simulink model "test_nncLKAsys"  (R2023a)
settings: Solver=VariableStepAuto  StartTime=0.0  StopTime=15  RelTol=1e-3
undefined symbols (not defined in the file): Cf, Cr, Iz, lf, lr, m, md, Ts, Vx
libraries: neural x49
(part 2 of 2)

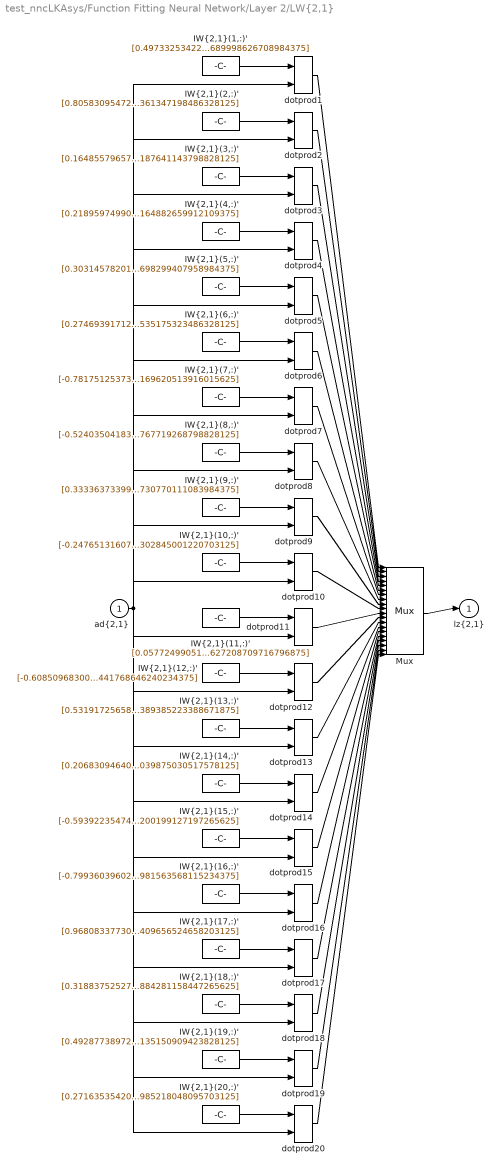
== system test_nncLKAsys/Function Fitting Neural Network/Layer 2/LW{2,1} ==
  "ad{2,1}" : Inport  PortDimensions=20
      mask Display: e = 0.06;c1 = [120 230 180]/255;c2 = ([120 230 180]+0)/(256+128);c3 = ([120 230 180]+128)/(256+128);patch([0 1 1 0],[0 0 1 1],c1);patch([0 1 1 1-e 1-e 0+e],[0 0 1 1-e 0+e 0+e],c2);patch([0 0 1 1-e 0+e 0+e],[0 1 1 1-e 1-e 0+e],c3);plot([0 1 1 0 0],[0 0 1 1 0]);
  "IW{2,1}(1,:)'" : Constant  Value=[0.4973325342225560774522818974219262599945068359375;0.90306464526148644278435995147447101771831512451171875;-0.496048746421447861454367966871359385550022125244140625;0.86588830289279539176305888759088702499866485595703125;0.258362950744856101348290167152299545705318450927734375;-0.7205856953057050429123364665429107844829559326171875;0.6406037637494745862198897157213650643825531005859375;0.054448589267391871160395311335378210060298442840576171875;0.05120315605558094229632359883908065967261791229248046875;0.734496230646326520030697793117724359035491943359375;0.440526641299326338074848763426416553556919097900390625;-0.443526764242088145095976869924925267696380615234375;-0.124610565537413064962635189658612944185733795166015625;0.495622454954692204243116293582716025412082672119140625;-0.274663451448240447660964491660706698894500732421875;-0.95942325063411926233669646535417996346950531005859375;-0.4074690282329813673101170934387482702732086181640625;-0.3830663272716934297790203345357440412044525146484375;0.37164147603418851151246826702845282852649688720703125;-0.418196849214901023028545523629873059689998626708984375]
      mask Display: e = 0.06;c1 = [120 150 230]/255;c2 = ([120 150 230]+0)/383;c3 = ([120 150 230]+128)/383;patch([0 1 1 0],[0 0 1 1],c1);patch([0 1 1 1-e 1-e 0+e],[0 0 1 1-e 0+e 0+e],c2);patch([0 0 1 1-e 0+e 0+e],[0 1 1 1-e 1-e 0+e],c3);plot([0 1 1 0 0],[0 0 1 1 0]);disp('weights');
  "IW{2,1}(10,:)'" : Constant  Value=[-0.2476513160780807465410902068470022641122341156005859375;-0.05048981524499081274814926700855721719563007354736328125;-0.83187777564385922968170916647068224847316741943359375;-0.1842943675353526378213331327060586772859096527099609375;-0.135408743923043306534026442022877745330333709716796875;0.213378955593828967263192453174269758164882659912109375;0.291693823371609373129587083894875831902027130126953125;-0.463136288082497682427884910794091410934925079345703125;-0.2209047101854656747210725598051794804632663726806640625;0.47999229837702539480659424953046254813671112060546875;0.70943574543465448556389674195088446140289306640625;-0.822960664207583736384776784689165651798248291015625;0.46371966171671552547906003383104689419269561767578125;0.35777426056320293934476239883224479854106903076171875;-0.053457236318613009229405719224814674817025661468505859375;-0.5644419341845097193299807258881628513336181640625;-0.830852975041227903574281299370341002941131591796875;-0.8407291227819257972697641889681108295917510986328125;-0.9051254349425936762685296343988738954067230224609375;-0.51676331967606270456627726161968894302845001220703125]
      mask Display: e = 0.06;c1 = [120 150 230]/255;c2 = ([120 150 230]+0)/383;c3 = ([120 150 230]+128)/383;patch([0 1 1 0],[0 0 1 1],c1);patch([0 1 1 1-e 1-e 0+e],[0 0 1 1-e 0+e 0+e],c2);patch([0 0 1 1-e 0+e 0+e],[0 1 1 1-e 1-e 0+e],c3);plot([0 1 1 0 0],[0 0 1 1 0]);disp('weights');
  "IW{2,1}(11,:)'" : Constant  Value=[0.057724990515373324206915839340581442229449748992919921875;-0.454959352688771134776146709555177949368953704833984375;0.686013523400408331553990137763321399688720703125;0.77761666694430864321674334860290400683879852294921875;-0.67233436458554962644740271571208722889423370361328125;0.262387251003185772990633495282963849604129791259765625;0.66393479253179810140039762700325809419155120849609375;-0.54205992204004826984231613096198998391628265380859375;0.659601736923068671103465021587908267974853515625;0.59560282814388243455283600269467569887638092041015625;-0.67025312054929220284549273856100626289844512939453125;-0.0109594114292667112187107392173857078887522220611572265625;0.1323308886400174078090685725328512489795684814453125;0.77709052240416143231271917102276347577571868896484375;-0.272148319240205383007236150660901330411434173583984375;0.59914332019493798942022522169281728565692901611328125;0.99457188770306415026567492532194592058658599853515625;0.37686351449791433143587937593110837042331695556640625;0.616532923458239512370937518426217138767242431640625;-0.3508767302809150390174863787251524627208709716796875]
      mask Display: e = 0.06;c1 = [120 150 230]/255;c2 = ([120 150 230]+0)/383;c3 = ([120 150 230]+128)/383;patch([0 1 1 0],[0 0 1 1],c1);patch([0 1 1 1-e 1-e 0+e],[0 0 1 1-e 0+e 0+e],c2);patch([0 0 1 1-e 0+e 0+e],[0 1 1 1-e 1-e 0+e],c3);plot([0 1 1 0 0],[0 0 1 1 0]);disp('weights');
  "IW{2,1}(12,:)'" : Constant  Value=[-0.60850968300268626354210255158250220119953155517578125;-0.65439626701131403674338571363477967679500579833984375;0.402047200135600302228766622647526673972606658935546875;0.3978796710819414439441743525094352662563323974609375;0.36291812080822760666620752090238966047763824462890625;0.4909388105689107550944072499987669289112091064453125;-0.480859970862364261012800170647096820175647735595703125;0.26633703325919200199933811745722778141498565673828125;-0.67734265099850732294584076953469775617122650146484375;-0.246990874667310122969610119980643503367900848388671875;-0.0149495709028309962940195276814847602508962154388427734375;0.85590287991131053235704939652350731194019317626953125;-0.52043442213506352356233719547162763774394989013671875;-0.72331221909417309223755410130252130329608917236328125;-0.72319113937276202630499710721778683364391326904296875;0.27801325599222603823790223032119683921337127685546875;-0.720583773337928779056937855784781277179718017578125;0.7117053121012466565531440210179425776004791259765625;0.19320449486644986070160712188226170837879180908203125;-0.55058864749936853311140794176026247441768646240234375]
      mask Display: e = 0.06;c1 = [120 150 230]/255;c2 = ([120 150 230]+0)/383;c3 = ([120 150 230]+128)/383;patch([0 1 1 0],[0 0 1 1],c1);patch([0 1 1 1-e 1-e 0+e],[0 0 1 1-e 0+e 0+e],c2);patch([0 0 1 1-e 0+e 0+e],[0 1 1 1-e 1-e 0+e],c3);plot([0 1 1 0 0],[0 0 1 1 0]);disp('weights');
  "IW{2,1}(13,:)'" : Constant  Value=[0.53191725658587396541321368204080499708652496337890625;-0.5684191622120613462953997441218234598636627197265625;0.21829186796840016615561808066559024155139923095703125;0.8434716025869997135799849274917505681514739990234375;-0.429187862165322064900152554400847293436527252197265625;-0.61841840572703576928148549995967186987400054931640625;0.6095584518567715992531930169207043945789337158203125;-0.276179360087225822528722574134008027613162994384765625;0.2433613583566199556340592380365706048905849456787109375;0.98001673052718574208341806297539733350276947021484375;-0.45880540181842321967309317187755368649959564208984375;0.06691757909025740358455180967212072573602199554443359375;-0.7740737648085611599668709459365345537662506103515625;0.8386821929981544965215789488865993916988372802734375;-0.76226447852808776328714657211094163358211517333984375;0.5511304110054016103248386571067385375499725341796875;0.239317115231703070321600534953176975250244140625;-0.75148183567851145614469032807392068207263946533203125;-0.475776517023930589633806675919913686811923980712890625;-0.65629454419391464181643414121936075389385223388671875]
      mask Display: e = 0.06;c1 = [120 150 230]/255;c2 = ([120 150 230]+0)/383;c3 = ([120 150 230]+128)/383;patch([0 1 1 0],[0 0 1 1],c1);patch([0 1 1 1-e 1-e 0+e],[0 0 1 1-e 0+e 0+e],c2);patch([0 0 1 1-e 0+e 0+e],[0 1 1 1-e 1-e 0+e],c3);plot([0 1 1 0 0],[0 0 1 1 0]);disp('weights');
  "IW{2,1}(14,:)'" : Constant  Value=[0.2068309464048300461147533724215463735163211822509765625;-0.060874669609953351023801104702215525321662425994873046875;0.042469111138720129494661392755006090737879276275634765625;0.75101380689437513549222558140172623097896575927734375;-0.2301884916521317325788231755723245441913604736328125;-0.64214453268418092424241194748901762068271636962890625;-0.37040855858182430981884181164787150919437408447265625;-0.70737191728260040424203225484234280884265899658203125;-0.135073111944455648281149251488386653363704681396484375;1.0030017572738476605564983401563949882984161376953125;0.554473075215879962485132637084461748600006103515625;-0.5767995535584378163918017889955081045627593994140625;-0.10154501148795087861476105217661825008690357208251953125;0.83011392912038461933121880065300501883029937744140625;-0.022470298944575924082744933230060269124805927276611328125;0.484985641342478512871849716248107142746448516845703125;-0.1963460027903477234101359272244735620915889739990234375;-0.261489162470172953334213161724619567394256591796875;0.88801671382668134757665256984182633459568023681640625;0.8012075193285348451155414295499213039875030517578125]
      mask Display: e = 0.06;c1 = [120 150 230]/255;c2 = ([120 150 230]+0)/383;c3 = ([120 150 230]+128)/383;patch([0 1 1 0],[0 0 1 1],c1);patch([0 1 1 1-e 1-e 0+e],[0 0 1 1-e 0+e 0+e],c2);patch([0 0 1 1-e 0+e 0+e],[0 1 1 1-e 1-e 0+e],c3);plot([0 1 1 0 0],[0 0 1 1 0]);disp('weights');
  "IW{2,1}(15,:)'" : Constant  Value=[-0.59392235474925125782164059273782186210155487060546875;0.2469970517320487501944370478668133728206157684326171875;-0.479182699839034775823876088907127268612384796142578125;-0.7565554149826076990592582660610787570476531982421875;-0.147267538182649870837082062280387617647647857666015625;-1.101355612636625291855807518004439771175384521484375;0.414661477953157830977914954928564839065074920654296875;-0.57924333285030626949918541868100874125957489013671875;-0.2822483427932775956747946111136116087436676025390625;0.365463041905304153456057747462182305753231048583984375;0.691449731034453396461003649164922535419464111328125;-0.484014696014661460754524568983470089733600616455078125;-0.3214298163255582263531096032238565385341644287109375;-0.2446932497166434961055614394354051910340785980224609375;0.87806342417053884208399949784507043659687042236328125;-0.6837950072062544126794136900571174919605255126953125;-0.1294637551593125490700941782051813788712024688720703125;-0.51639178539500318887434104908606968820095062255859375;-0.8628656967513392839208563600550405681133270263671875;0.57210024503377587823393923827097751200199127197265625]
      mask Display: e = 0.06;c1 = [120 150 230]/255;c2 = ([120 150 230]+0)/383;c3 = ([120 150 230]+128)/383;patch([0 1 1 0],[0 0 1 1],c1);patch([0 1 1 1-e 1-e 0+e],[0 0 1 1-e 0+e 0+e],c2);patch([0 0 1 1-e 0+e 0+e],[0 1 1 1-e 1-e 0+e],c3);plot([0 1 1 0 0],[0 0 1 1 0]);disp('weights');
  "IW{2,1}(16,:)'" : Constant  Value=[-0.79936039602108255319734553268062882125377655029296875;-0.9038848231317271331164420189452357590198516845703125;0.404706321969310167663280708438833244144916534423828125;0.369308486120014212161777322762645781040191650390625;-0.73588945289850615782967224731692112982273101806640625;0.2109720089806362552931062737116008065640926361083984375;0.80563130849964437185661836338113062083721160888671875;0.173851749513278586167785988436662591993808746337890625;-0.2151500541783762654457490270942798815667629241943359375;0.408657702026222369173780180062749423086643218994140625;-0.9027615049856836382247138317325152456760406494140625;0.0172054680890415361005363337199014495126903057098388671875;-0.8622846305143279099780784235917963087558746337890625;-0.51387189745748995672869341433397494256496429443359375;-0.55544867935312336459929838383686728775501251220703125;0.3756122611517251907997660964610986411571502685546875;0.553092246700364942313399296835996210575103759765625;-0.84888335556626592914852835747296921908855438232421875;-0.8758198815178668272807271932833828032016754150390625;0.74301445501374396851446135769947431981563568115234375]
      mask Display: e = 0.06;c1 = [120 150 230]/255;c2 = ([120 150 230]+0)/383;c3 = ([120 150 230]+128)/383;patch([0 1 1 0],[0 0 1 1],c1);patch([0 1 1 1-e 1-e 0+e],[0 0 1 1-e 0+e 0+e],c2);patch([0 0 1 1-e 0+e 0+e],[0 1 1 1-e 1-e 0+e],c3);plot([0 1 1 0 0],[0 0 1 1 0]);disp('weights');
  "IW{2,1}(17,:)'" : Constant  Value=[0.96808337730736437887202328056446276605129241943359375;0.8804707813004741812079601004370488226413726806640625;0.102363658179670580228304288539220578968524932861328125;-0.8352226572803538306999371343408711254596710205078125;0.9505108042221801500915034921490587294101715087890625;0.438235898788289002236950864244136027991771697998046875;0.38577234970647855671899151275283657014369964599609375;-0.1208143097052460090967684891438693739473819732666015625;-0.77150614240208081895389113924466073513031005859375;0.84947514259350132004300348853575997054576873779296875;-0.1487735383250336218541320931763038970530033111572265625;0.87542171746614150240617391318664886057376861572265625;-0.94090955821116850632535033582826144993305206298828125;-0.89715669844669954091642694038455374538898468017578125;-0.81592915906335949927097317413426935672760009765625;0.492156990589912857192445017062709666788578033447265625;0.08283113566716497622177683979316498152911663055419921875;-0.488791100114578214164140490538557060062885284423828125;0.2348206770858200786999958609158056788146495819091796875;0.59500478527796485384016023090225644409656524658203125]
      mask Display: e = 0.06;c1 = [120 150 230]/255;c2 = ([120 150 230]+0)/383;c3 = ([120 150 230]+128)/383;patch([0 1 1 0],[0 0 1 1],c1);patch([0 1 1 1-e 1-e 0+e],[0 0 1 1-e 0+e 0+e],c2);patch([0 0 1 1-e 0+e 0+e],[0 1 1 1-e 1-e 0+e],c3);plot([0 1 1 0 0],[0 0 1 1 0]);disp('weights');
  "IW{2,1}(18,:)'" : Constant  Value=[0.318837525273336808151469767835806123912334442138671875;-0.0466292350120939003144115986287943087518215179443359375;0.74492191849115896307154116584570147097110748291015625;1.0461389061517232246245612259372137486934661865234375;0.8703366566824921601863707110169343650341033935546875;0.807666727616154656033131686854176223278045654296875;-0.79258773942038052151559668345726095139980316162109375;0.00021271701060131438520972579908629995770752429962158203125;0.811323814918487595804208467598073184490203857421875;-0.8942994208564523095361664672964252531528472900390625;0.704688427044971366086656416882760822772979736328125;-1.0132738674596739603117612205096520483493804931640625;0.30231916343964126969723338334006257355213165283203125;0.81174905074590653075716772946179844439029693603515625;-0.0025264614549911266171144941239390391274355351924896240234375;-0.33930147473698590854240819680853746831417083740234375;-0.1348439869058445095273413016911945305764675140380859375;-0.60934272120341559375589213232160545885562896728515625;0.94357254222468689430769472892279736697673797607421875;-0.83417721244480935727239057086990214884281158447265625]
      mask Display: e = 0.06;c1 = [120 150 230]/255;c2 = ([120 150 230]+0)/383;c3 = ([120 150 230]+128)/383;patch([0 1 1 0],[0 0 1 1],c1);patch([0 1 1 1-e 1-e 0+e],[0 0 1 1-e 0+e 0+e],c2);patch([0 0 1 1-e 0+e 0+e],[0 1 1 1-e 1-e 0+e],c3);plot([0 1 1 0 0],[0 0 1 1 0]);disp('weights');
  "IW{2,1}(19,:)'" : Constant  Value=[0.492877389721817438239526154575287364423274993896484375;-0.0923419800480494712413559454944333992898464202880859375;-0.74935841359499388847353884557378478348255157470703125;0.576589450600195174700957068125717341899871826171875;-0.99791744673630156103882882234756834805011749267578125;-0.73787636620029173339929684516391716897487640380859375;0.01722967903821918944640145809898967854678630828857421875;0.76265477713131069048557719725067727267742156982421875;-0.6305833473085218354725611789035610854625701904296875;-0.25163934565438650370339246364892460405826568603515625;-0.30769952527755373150597506537451408803462982177734375;-0.776728817612701849526501973741687834262847900390625;-0.299691123768055955878253371338360011577606201171875;0.26263947903921580628860965589410625398159027099609375;-0.412400257488821642137821754658943973481655120849609375;-0.631856264616108997955734594142995774745941162109375;-1.025930891543680889554934765328653156757354736328125;0.1727106956326584230598797375932917930185794830322265625;-0.704919595179296809561719783232547342777252197265625;-0.6960369704409388180721407479722984135150909423828125]
      mask Display: e = 0.06;c1 = [120 150 230]/255;c2 = ([120 150 230]+0)/383;c3 = ([120 150 230]+128)/383;patch([0 1 1 0],[0 0 1 1],c1);patch([0 1 1 1-e 1-e 0+e],[0 0 1 1-e 0+e 0+e],c2);patch([0 0 1 1-e 0+e 0+e],[0 1 1 1-e 1-e 0+e],c3);plot([0 1 1 0 0],[0 0 1 1 0]);disp('weights');
  "IW{2,1}(2,:)'" : Constant  Value=[0.80583095472733867747905378564610145986080169677734375;-0.5040439751989380656738148900330998003482818603515625;0.49076548759692217860362006831564940512180328369140625;-0.2836617428346477343126252890215255320072174072265625;-0.32930254071776421387340860746917314827442169189453125;0.6782881784273981917721130230347625911235809326171875;0.025643782612106112706040761395342997275292873382568359375;-0.85777680483196572236437305036815814673900604248046875;-0.8852900683144795390688841507653705775737762451171875;-0.43402105081971920075289972373866476118564605712890625;0.69030295362972660111466893795295618474483489990234375;-0.419727830953746827713501943435403518378734588623046875;-0.26175127499150629972746173734776675701141357421875;0.21829284731629317040102478131302632391452789306640625;0.73264701286658018286601645741029642522335052490234375;-0.51866922709361429344454563761246390640735626220703125;-0.2065670486297002117481724781100638210773468017578125;-0.175588234770689133323884334458853118121623992919921875;0.71154748838845449654399999417364597320556640625;-0.73510468819661867190262682925094850361347198486328125]
      mask Display: e = 0.06;c1 = [120 150 230]/255;c2 = ([120 150 230]+0)/383;c3 = ([120 150 230]+128)/383;patch([0 1 1 0],[0 0 1 1],c1);patch([0 1 1 1-e 1-e 0+e],[0 0 1 1-e 0+e 0+e],c2);patch([0 0 1 1-e 0+e 0+e],[0 1 1 1-e 1-e 0+e],c3);plot([0 1 1 0 0],[0 0 1 1 0]);disp('weights');
  "IW{2,1}(20,:)'" : Constant  Value=[0.271635354201527456918796588070108555257320404052734375;0.54318743882764319863554192124865949153900146484375;0.7223971884144599897581429104320704936981201171875;-0.49056572301568868166299353106296621263027191162109375;-0.0104319287920506820199761932599358260631561279296875;-0.04014657611138956749829986847544205375015735626220703125;0.55120095340672670136683564123813994228839874267578125;-0.98412206709895644340946319061913527548313140869140625;0.7648118130093648492362490287632681429386138916015625;0.58356460622945516281134814562392421066761016845703125;-0.68452778429240301871772089725709520280361175537109375;-0.77895939407926906294932223318028263747692108154296875;-0.550984972152189556027224170975387096405029296875;0.2158209808063560053437157648659194819629192352294921875;0.53414817491611688016206471729674376547336578369140625;0.12220956823076724317989061319167376495897769927978515625;-0.41618577872106954362863007190753705799579620361328125;0.73268368804328110055479328366345725953578948974609375;-0.2200058204088935764897172475684783421456813812255859375;-0.9676238535067736012962313907337374985218048095703125]
      mask Display: e = 0.06;c1 = [120 150 230]/255;c2 = ([120 150 230]+0)/383;c3 = ([120 150 230]+128)/383;patch([0 1 1 0],[0 0 1 1],c1);patch([0 1 1 1-e 1-e 0+e],[0 0 1 1-e 0+e 0+e],c2);patch([0 0 1 1-e 0+e 0+e],[0 1 1 1-e 1-e 0+e],c3);plot([0 1 1 0 0],[0 0 1 1 0]);disp('weights');
  "IW{2,1}(3,:)'" : Constant  Value=[0.1648557965756184129357819756478420458734035491943359375;-0.378070860144959441928591559189953841269016265869140625;-0.4454647788033614386193903555977158248424530029296875;-0.52065178472906270545905726976343430578708648681640625;0.2190857779921936698830364775858470238745212554931640625;0.79944556312198800096524564651190303266048431396484375;-0.1724478535534694489950169327130424790084362030029296875;0.354602901326104114065884687079233117401599884033203125;-0.25039973585231967145858789081103168427944183349609375;-0.92375174374951607436656786376261152327060699462890625;-1.009033751754920604781773363356478512287139892578125;0.53110251050317913712461859176983125507831573486328125;0.60084665244582124987715587849379517138004302978515625;0.53112732155433761693785754687269218266010284423828125;-0.87803964804421641421328104115673340857028961181640625;0.28242671580565270605944760973216034471988677978515625;-0.40495162503179338298053835387690924108028411865234375;-0.57440279853582421054625228862278163433074951171875;0.698851098380761204253985852119512856006622314453125;-0.235177470414115408203770130057819187641143798828125]
      mask Display: e = 0.06;c1 = [120 150 230]/255;c2 = ([120 150 230]+0)/383;c3 = ([120 150 230]+128)/383;patch([0 1 1 0],[0 0 1 1],c1);patch([0 1 1 1-e 1-e 0+e],[0 0 1 1-e 0+e 0+e],c2);patch([0 0 1 1-e 0+e 0+e],[0 1 1 1-e 1-e 0+e],c3);plot([0 1 1 0 0],[0 0 1 1 0]);disp('weights');
  "IW{2,1}(4,:)'" : Constant  Value=[0.21895974990214739364091656170785427093505859375;0.10759463660579758614854739562360919080674648284912109375;-0.8830983651156909530755001469515264034271240234375;0.00084012421230144772484049742189426979166455566883087158203125;0.0348551728222384060718042064763722009956836700439453125;0.1924257232616762014476563535936293192207813262939453125;-0.0814550600676816893841447608792805112898349761962890625;-0.2029207728504890673182359250859008170664310455322265625;0.01120949158410411601594081076882503111846745014190673828125;0.07517792203270250162017163120253826491534709930419921875;0.88448504942889683011486567920655943453311920166015625;-0.15189814262597700622592356012319214642047882080078125;-0.67528631620519730116569689926109276711940765380859375;0.200299015937956514932238860637880861759185791015625;-0.60042380325334543389459440732025541365146636962890625;-0.59445463786334562517055246644304133951663970947265625;-0.481983452535620748857780881735379807651042938232421875;0.3326420580904938528732373015373013913631439208984375;-0.93253094455460028289195406614453531801700592041015625;-0.3893884834864100863427438525832258164882659912109375]
      mask Display: e = 0.06;c1 = [120 150 230]/255;c2 = ([120 150 230]+0)/383;c3 = ([120 150 230]+128)/383;patch([0 1 1 0],[0 0 1 1],c1);patch([0 1 1 1-e 1-e 0+e],[0 0 1 1-e 0+e 0+e],c2);patch([0 0 1 1-e 0+e 0+e],[0 1 1 1-e 1-e 0+e],c3);plot([0 1 1 0 0],[0 0 1 1 0]);disp('weights');
  "IW{2,1}(5,:)'" : Constant  Value=[0.303145782014597298115177181898616254329681396484375;0.96289211952739861555272682380746118724346160888671875;0.2115476781969203579070182286159251816570758819580078125;-0.032281579539018494251489954649514402262866497039794921875;0.54695371368049061633342944332980550825595855712890625;-0.258860133802492564658592755222343839704990386962890625;-0.286501970669331085250775004169554449617862701416015625;-1.02229993603627189457938584382645785808563232421875;-0.5243286007645371338270479100174270570278167724609375;0.5682424154315814934790296319988556206226348876953125;0.263940691667868154723919360549189150333404541015625;0.73496117657963677682886327602318488061428070068359375;0.437762223225590274555685255108983255922794342041015625;0.49665425185079736802862271360936574637889862060546875;0.79653836625578311458895086616394110023975372314453125;0.94338790284457640922255450277589261531829833984375;-1.0605684469712344242253720949520356953144073486328125;-0.337327559909715635200200267718173563480377197265625;-0.284806816810242613424719593240297399461269378662109375;0.67511261727602744908693921388476155698299407958984375]
      mask Display: e = 0.06;c1 = [120 150 230]/255;c2 = ([120 150 230]+0)/383;c3 = ([120 150 230]+128)/383;patch([0 1 1 0],[0 0 1 1],c1);patch([0 1 1 1-e 1-e 0+e],[0 0 1 1-e 0+e 0+e],c2);patch([0 0 1 1-e 0+e 0+e],[0 1 1 1-e 1-e 0+e],c3);plot([0 1 1 0 0],[0 0 1 1 0]);disp('weights');
  "IW{2,1}(6,:)'" : Constant  Value=[0.274693917128629949697682377518503926694393157958984375;-0.54256172182784834223667758124065585434436798095703125;-0.2299161652186730575575523971565417014062404632568359375;-0.7367689078729384721810902192373760044574737548828125;0.040915595850013551648682863515205099247395992279052734375;-0.2864715945795899276760110296891070902347564697265625;0.1051665936899386644132192714096163399517536163330078125;0.3249791110710342767475822256528772413730621337890625;-0.1326893109012770854970852951737469993531703948974609375;0.43832447660876550088460135157220065593719482421875;1.0372596204346582471345072917756624519824981689453125;-0.049182115345159170549660387905532843433320522308349609375;0.1136224075494485508119879568766918964684009552001953125;0.74712614037188107563025596391526050865650177001953125;-0.60080007047927741492543418644345365464687347412109375;0.5564611481820131988484945395612157881259918212890625;-0.33861233802811085968897941711475141346454620361328125;-0.5929495239255972993674959070631302893161773681640625;-0.8963266806159617683391616083099506795406341552734375;0.59191934379636734764318362067569978535175323486328125]
      mask Display: e = 0.06;c1 = [120 150 230]/255;c2 = ([120 150 230]+0)/383;c3 = ([120 150 230]+128)/383;patch([0 1 1 0],[0 0 1 1],c1);patch([0 1 1 1-e 1-e 0+e],[0 0 1 1-e 0+e 0+e],c2);patch([0 0 1 1-e 0+e 0+e],[0 1 1 1-e 1-e 0+e],c3);plot([0 1 1 0 0],[0 0 1 1 0]);disp('weights');
  "IW{2,1}(7,:)'" : Constant  Value=[-0.78175125373027098962808167925686575472354888916015625;0.04586908372922766929935534108153660781681537628173828125;0.65030567246522341662284816266037523746490478515625;0.768120239997597042957977464538998901844024658203125;-0.66196428473080171084319545116159133613109588623046875;0.43524619828663257958822896398487500846385955810546875;0.1354553386052981256426619438570924103260040283203125;-0.0285309870483352982784008844419076922349631786346435546875;0.1635635501616755360654309470191947184503078460693359375;-0.409127925620531407435720439025317318737506866455078125;-0.1451357321621767615393849837346351705491542816162109375;-0.086908773762445379329477646024315617978572845458984375;0.54818759080923629145587483435519970953464508056640625;-0.770635622273359022216254743398167192935943603515625;-0.7235665918684606179311913365381769835948944091796875;-0.343067390907107305775269878722610883414745330810546875;0.376987319150801580835974391447962261736392974853515625;-0.6913541405599676892279603634960949420928955078125;0.287418853966744103356489858924760483205318450927734375;0.28025767887580654846857441953034140169620513916015625]
      mask Display: e = 0.06;c1 = [120 150 230]/255;c2 = ([120 150 230]+0)/383;c3 = ([120 150 230]+128)/383;patch([0 1 1 0],[0 0 1 1],c1);patch([0 1 1 1-e 1-e 0+e],[0 0 1 1-e 0+e 0+e],c2);patch([0 0 1 1-e 0+e 0+e],[0 1 1 1-e 1-e 0+e],c3);plot([0 1 1 0 0],[0 0 1 1 0]);disp('weights');
  "IW{2,1}(8,:)'" : Constant  Value=[-0.5240350418371433338649012512178160250186920166015625;0.1468032595432306741667360938663478009402751922607421875;-0.8963773563722090553795851519680581986904144287109375;-0.18453196118392778402039766660891473293304443359375;0.026108014553306323202175320830065174959599971771240234375;0.3311305255037246819682650311733596026897430419921875;-0.6286305690971756288121241595945321023464202880859375;0.9102780907379008912272411180310882627964019775390625;0.42188122194594657177191265873261727392673492431640625;-0.4318229542546461185992257014731876552104949951171875;0.239711609026535155120285480734310112893581390380859375;0.193728712325672958183275795818190090358257293701171875;0.1864043574825079152557094630537903867661952972412109375;0.50061752598828890281623671398847363889217376708984375;0.55615866240797640074333685333840548992156982421875;0.1145172345983924422352373539979453198611736297607421875;0.038126489553497573681273280499226530082523822784423828125;0.319397937306894252884603702113963663578033447265625;-0.5350561036251908486605088910437189042568206787109375;0.115078445787836713964935597687144763767719268798828125]
      mask Display: e = 0.06;c1 = [120 150 230]/255;c2 = ([120 150 230]+0)/383;c3 = ([120 150 230]+128)/383;patch([0 1 1 0],[0 0 1 1],c1);patch([0 1 1 1-e 1-e 0+e],[0 0 1 1-e 0+e 0+e],c2);patch([0 0 1 1-e 0+e 0+e],[0 1 1 1-e 1-e 0+e],c3);plot([0 1 1 0 0],[0 0 1 1 0]);disp('weights');
  "IW{2,1}(9,:)'" : Constant  Value=[0.33336373399976138021116867093951441347599029541015625;-0.0778437448674461907049959563664742745459079742431640625;0.78101119215755498981224036469939164817333221435546875;0.231763459963500173532935377807007171213626861572265625;0.66849423146913211635222751283436082303524017333984375;-0.851409495772368796195905815693549811840057373046875;0.356976698538490844203607821327750571072101593017578125;-0.20337232270345506623954179303837008774280548095703125;0.84994959546992177035207305380026809871196746826171875;-0.342522901926370082481554391051759012043476104736328125;0.1383260727915899546136557773934327997267246246337890625;-0.016753345873249218811462668554668198339641094207763671875;0.375366583455239821720539339366951026022434234619140625;-0.87862942553470946283056264292099513113498687744140625;0.443086475898577691889812513181823305785655975341796875;-0.025102269902763284237234842066754936240613460540771484375;0.81368693872160668956183826594497077167034149169921875;-0.314434032118331263649935181092587299644947052001953125;-0.09779106365816823964731696605667821131646633148193359375;-0.50076148290063515755576872834353707730770111083984375]
      mask Display: e = 0.06;c1 = [120 150 230]/255;c2 = ([120 150 230]+0)/383;c3 = ([120 150 230]+128)/383;patch([0 1 1 0],[0 0 1 1],c1);patch([0 1 1 1-e 1-e 0+e],[0 0 1 1-e 0+e 0+e],c2);patch([0 0 1 1-e 0+e 0+e],[0 1 1 1-e 1-e 0+e],c3);plot([0 1 1 0 0],[0 0 1 1 0]);disp('weights');
  Mux : Mux  Inputs=20
      mask Display: e = 0.06;c1 = [120 150 230]/255;c2 = ([120 150 230]+0)/383;c3 = ([120 150 230]+128)/383;patch([0 1 1 0],[0 0 1 1],c1);patch([0 1 1 1-e 1-e 0+e],[0 0 1 1-e 0+e 0+e],c2);patch([0 0 1 1-e 0+e 0+e],[0 1 1 1-e 1-e 0+e],c3);plot([0 1 1 0 0],[0 0 1 1 0]);disp('Mux');
  dotprod{1..20} (20 alike) : neural/Weight Functions/dotprod
  "lz{2,1}" : Outport
      mask Display: e = 0.06;c1 = [120 230 180]/255;c2 = ([120 230 180]+0)/(256+128);c3 = ([120 230 180]+128)/(256+128);patch([0 1 1 0],[0 0 1 1],c1);patch([0 1 1 1-e 1-e 0+e],[0 0 1 1-e 0+e 0+e],c2);patch([0 0 1 1-e 0+e 0+e],[0 1 1 1-e 1-e 0+e],c3);plot([0 1 1 0 0],[0 0 1 1 0]);
  wires:
  "IW{2,1}(1,:)'"/1 -> dotprod1/1
  "ad{2,1}"/1 -> dotprod1/2, dotprod2/2, dotprod3/2, dotprod4/2, dotprod5/2, dotprod6/2, dotprod7/2, dotprod8/2, dotprod9/2, dotprod10/2, dotprod11/2, dotprod12/2, dotprod13/2, dotprod14/2, dotprod15/2, dotprod16/2, dotprod17/2, dotprod18/2, dotprod19/2, dotprod20/2
  dotprod1/1 -> Mux/1
  "IW{2,1}(2,:)'"/1 -> dotprod2/1
  dotprod2/1 -> Mux/2
  "IW{2,1}(3,:)'"/1 -> dotprod3/1
  dotprod3/1 -> Mux/3
  "IW{2,1}(4,:)'"/1 -> dotprod4/1
  dotprod4/1 -> Mux/4
  "IW{2,1}(5,:)'"/1 -> dotprod5/1
  dotprod5/1 -> Mux/5
  "IW{2,1}(6,:)'"/1 -> dotprod6/1
  dotprod6/1 -> Mux/6
  "IW{2,1}(7,:)'"/1 -> dotprod7/1
  dotprod7/1 -> Mux/7
  "IW{2,1}(8,:)'"/1 -> dotprod8/1
  dotprod8/1 -> Mux/8
  "IW{2,1}(9,:)'"/1 -> dotprod9/1
  dotprod9/1 -> Mux/9
  "IW{2,1}(10,:)'"/1 -> dotprod10/1
  dotprod10/1 -> Mux/10
  "IW{2,1}(11,:)'"/1 -> dotprod11/1
  dotprod11/1 -> Mux/11
  "IW{2,1}(12,:)'"/1 -> dotprod12/1
  dotprod12/1 -> Mux/12
  "IW{2,1}(13,:)'"/1 -> dotprod13/1
  dotprod13/1 -> Mux/13
  "IW{2,1}(14,:)'"/1 -> dotprod14/1
  dotprod14/1 -> Mux/14
  "IW{2,1}(15,:)'"/1 -> dotprod15/1
  dotprod15/1 -> Mux/15
  "IW{2,1}(16,:)'"/1 -> dotprod16/1
  dotprod16/1 -> Mux/16
  "IW{2,1}(17,:)'"/1 -> dotprod17/1
  dotprod17/1 -> Mux/17
  "IW{2,1}(18,:)'"/1 -> dotprod18/1
  dotprod18/1 -> Mux/18
  "IW{2,1}(19,:)'"/1 -> dotprod19/1
  dotprod19/1 -> Mux/19
  "IW{2,1}(20,:)'"/1 -> dotprod20/1
  dotprod20/1 -> Mux/20
  Mux/1 -> "lz{2,1}"/1

== system test_nncLKAsys/Function Fitting Neural Network/Layer 3/Delays 1 ==
  "p{3}" : Inport  PortDimensions=20
      mask Display: e = 0.06;c1 = [120 230 180]/255;c2 = ([120 230 180]+0)/(256+128);c3 = ([120 230 180]+128)/(256+128);patch([0 1 1 0],[0 0 1 1],c1);patch([0 1 1 1-e 1-e 0+e],[0 0 1 1-e 0+e 0+e],c2);patch([0 0 1 1-e 0+e 0+e],[0 1 1 1-e 1-e 0+e],c3);plot([0 1 1 0 0],[0 0 1 1 0]);
  mux : Mux  Inputs=1
      mask Display: e = 0.06;c1 = [120 150 230]/255;c2 = ([120 150 230]+0)/383;c3 = ([120 150 230]+128)/383;patch([0 1 1 0],[0 0 1 1],c1);patch([0 1 1 1-e 1-e 0+e],[0 0 1 1-e 0+e 0+e],c2);patch([0 0 1 1-e 0+e 0+e],[0 1 1 1-e 1-e 0+e],c3);plot([0 1 1 0 0],[0 0 1 1 0]);disp('Mux')
  "pd{3,2}" : Outport
      mask Display: e = 0.06;c1 = [120 230 180]/255;c2 = ([120 230 180]+0)/(256+128);c3 = ([120 230 180]+128)/(256+128);patch([0 1 1 0],[0 0 1 1],c1);patch([0 1 1 1-e 1-e 0+e],[0 0 1 1-e 0+e 0+e],c2);patch([0 0 1 1-e 0+e 0+e],[0 1 1 1-e 1-e 0+e],c3);plot([0 1 1 0 0],[0 0 1 1 0]);
  wires:
  "p{3}"/1 -> mux/1
  mux/1 -> "pd{3,2}"/1

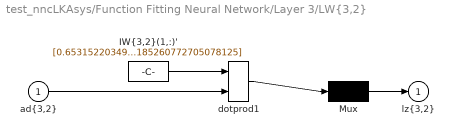
== system test_nncLKAsys/Function Fitting Neural Network/Layer 3/LW{3,2} ==
  "ad{3,2}" : Inport  PortDimensions=20
      mask Display: e = 0.06;c1 = [120 230 180]/255;c2 = ([120 230 180]+0)/(256+128);c3 = ([120 230 180]+128)/(256+128);patch([0 1 1 0],[0 0 1 1],c1);patch([0 1 1 1-e 1-e 0+e],[0 0 1 1-e 0+e 0+e],c2);patch([0 0 1 1-e 0+e 0+e],[0 1 1 1-e 1-e 0+e],c3);plot([0 1 1 0 0],[0 0 1 1 0]);
  "IW{3,2}(1,:)'" : Constant  Value=[0.65315220349572788993697258774773217737674713134765625;0.29344964644723925406566422680043615400791168212890625;-0.90542067539335746584328035169164650142192840576171875;-0.2403719112579951744379513911553658545017242431640625;-0.53273019691572986999972272315062582492828369140625;0.67291485788423965885840516421012580394744873046875;0.47338993780191651605804281643941067159175872802734375;0.072284909129924468373928903019987046718597412109375;0.7324026572186046468715403534588403999805450439453125;0.20374196992978366171911375204217620193958282470703125;0.5311078510055853296734085233765654265880584716796875;0.479381227700912460054638586370856501162052154541015625;0.478120958059007339358004173845984041690826416015625;0.7329036462281661723494607940665446221828460693359375;1.2501354768980752485418861397192813456058502197265625;-0.2298729992777493735811589203876792453229427337646484375;0.6088424086004555757511980118579231202602386474609375;-1.026894434446469883681629653437994420528411865234375;-0.91304088493900470435704619376338087022304534912109375;-0.83616715886671777457905818664585240185260772705078125]
      mask Display: e = 0.06;c1 = [120 150 230]/255;c2 = ([120 150 230]+0)/383;c3 = ([120 150 230]+128)/383;patch([0 1 1 0],[0 0 1 1],c1);patch([0 1 1 1-e 1-e 0+e],[0 0 1 1-e 0+e 0+e],c2);patch([0 0 1 1-e 0+e 0+e],[0 1 1 1-e 1-e 0+e],c3);plot([0 1 1 0 0],[0 0 1 1 0]);disp('weights');
  Mux : Mux  Inputs=1
      mask Display: e = 0.06;c1 = [120 150 230]/255;c2 = ([120 150 230]+0)/383;c3 = ([120 150 230]+128)/383;patch([0 1 1 0],[0 0 1 1],c1);patch([0 1 1 1-e 1-e 0+e],[0 0 1 1-e 0+e 0+e],c2);patch([0 0 1 1-e 0+e 0+e],[0 1 1 1-e 1-e 0+e],c3);plot([0 1 1 0 0],[0 0 1 1 0]);disp('Mux');
  dotprod1 : neural/Weight Functions/dotprod
  "lz{3,2}" : Outport
      mask Display: e = 0.06;c1 = [120 230 180]/255;c2 = ([120 230 180]+0)/(256+128);c3 = ([120 230 180]+128)/(256+128);patch([0 1 1 0],[0 0 1 1],c1);patch([0 1 1 1-e 1-e 0+e],[0 0 1 1-e 0+e 0+e],c2);patch([0 0 1 1-e 0+e 0+e],[0 1 1 1-e 1-e 0+e],c3);plot([0 1 1 0 0],[0 0 1 1 0]);
  wires:
  "IW{3,2}(1,:)'"/1 -> dotprod1/1
  "ad{3,2}"/1 -> dotprod1/2
  dotprod1/1 -> Mux/1
  Mux/1 -> "lz{3,2}"/1

== system test_nncLKAsys/Function Fitting Neural Network/Layer 4/Delays 1 ==
  "p{4}" : Inport  PortDimensions=1
      mask Display: e = 0.06;c1 = [120 230 180]/255;c2 = ([120 230 180]+0)/(256+128);c3 = ([120 230 180]+128)/(256+128);patch([0 1 1 0],[0 0 1 1],c1);patch([0 1 1 1-e 1-e 0+e],[0 0 1 1-e 0+e 0+e],c2);patch([0 0 1 1-e 0+e 0+e],[0 1 1 1-e 1-e 0+e],c3);plot([0 1 1 0 0],[0 0 1 1 0]);
  mux : Mux  Inputs=1
      mask Display: e = 0.06;c1 = [120 150 230]/255;c2 = ([120 150 230]+0)/383;c3 = ([120 150 230]+128)/383;patch([0 1 1 0],[0 0 1 1],c1);patch([0 1 1 1-e 1-e 0+e],[0 0 1 1-e 0+e 0+e],c2);patch([0 0 1 1-e 0+e 0+e],[0 1 1 1-e 1-e 0+e],c3);plot([0 1 1 0 0],[0 0 1 1 0]);disp('Mux')
  "pd{4,3}" : Outport
      mask Display: e = 0.06;c1 = [120 230 180]/255;c2 = ([120 230 180]+0)/(256+128);c3 = ([120 230 180]+128)/(256+128);patch([0 1 1 0],[0 0 1 1],c1);patch([0 1 1 1-e 1-e 0+e],[0 0 1 1-e 0+e 0+e],c2);patch([0 0 1 1-e 0+e 0+e],[0 1 1 1-e 1-e 0+e],c3);plot([0 1 1 0 0],[0 0 1 1 0]);
  wires:
  "p{4}"/1 -> mux/1
  mux/1 -> "pd{4,3}"/1

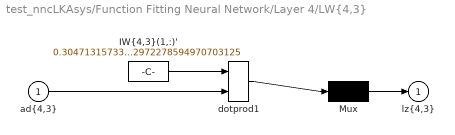
== system test_nncLKAsys/Function Fitting Neural Network/Layer 4/LW{4,3} ==
  "ad{4,3}" : Inport  PortDimensions=1
      mask Display: e = 0.06;c1 = [120 230 180]/255;c2 = ([120 230 180]+0)/(256+128);c3 = ([120 230 180]+128)/(256+128);patch([0 1 1 0],[0 0 1 1],c1);patch([0 1 1 1-e 1-e 0+e],[0 0 1 1-e 0+e 0+e],c2);patch([0 0 1 1-e 0+e 0+e],[0 1 1 1-e 1-e 0+e],c3);plot([0 1 1 0 0],[0 0 1 1 0]);
  "IW{4,3}(1,:)'" : Constant  Value=0.30471315733376880263705288598430342972278594970703125
      mask Display: e = 0.06;c1 = [120 150 230]/255;c2 = ([120 150 230]+0)/383;c3 = ([120 150 230]+128)/383;patch([0 1 1 0],[0 0 1 1],c1);patch([0 1 1 1-e 1-e 0+e],[0 0 1 1-e 0+e 0+e],c2);patch([0 0 1 1-e 0+e 0+e],[0 1 1 1-e 1-e 0+e],c3);plot([0 1 1 0 0],[0 0 1 1 0]);disp('weights');
  Mux : Mux  Inputs=1
      mask Display: e = 0.06;c1 = [120 150 230]/255;c2 = ([120 150 230]+0)/383;c3 = ([120 150 230]+128)/383;patch([0 1 1 0],[0 0 1 1],c1);patch([0 1 1 1-e 1-e 0+e],[0 0 1 1-e 0+e 0+e],c2);patch([0 0 1 1-e 0+e 0+e],[0 1 1 1-e 1-e 0+e],c3);plot([0 1 1 0 0],[0 0 1 1 0]);disp('Mux');
  dotprod1 : neural/Weight Functions/dotprod
  "lz{4,3}" : Outport
      mask Display: e = 0.06;c1 = [120 230 180]/255;c2 = ([120 230 180]+0)/(256+128);c3 = ([120 230 180]+128)/(256+128);patch([0 1 1 0],[0 0 1 1],c1);patch([0 1 1 1-e 1-e 0+e],[0 0 1 1-e 0+e 0+e],c2);patch([0 0 1 1-e 0+e 0+e],[0 1 1 1-e 1-e 0+e],c3);plot([0 1 1 0 0],[0 0 1 1 0]);
  wires:
  "IW{4,3}(1,:)'"/1 -> dotprod1/1
  "ad{4,3}"/1 -> dotprod1/2
  dotprod1/1 -> Mux/1
  Mux/1 -> "lz{4,3}"/1

== matlab function test_nncLKAsys/Curvature Previewer/MATLAB Function ==
  settings: updateMethod=DISCRETE  sampleTime=ts
  data: data parameter; seq output; steps parameter; t input; first output; next_t output
function [seq,first,next_t] = fcn(data,steps,t)
%#codegen
[seq,first,next_t] = mpcblock_preview('md',data,steps,t);
